simulink model "pruebaSimulink"  (Simulink 7.1)
settings: Solver=ode45  StartTime=0.0  StopTime=5  RelTol=1e-3
libraries: dsparch4 x1
settings Model: Creator=Usuario  LastModifiedBy=Usuario

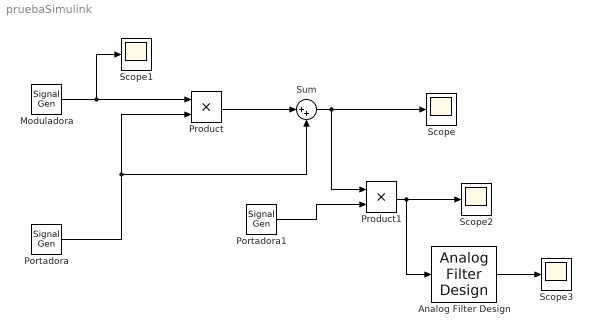
== system pruebaSimulink ==
  Analog Filter Design : dsparch4/Analog Filter Design  method=Butterworth  filttype=Lowpass  N=8  Wlo=30  Whi=80  Rp=2  Rs=40
  Moduladora : SignalGenerator
  Portadora : SignalGenerator  Frequency=10
  Portadora1 : SignalGenerator  Frequency=10
  Product : Product  OutDataType=sfix(16)  OutScaling=2^0  SampleTime=0.001  RndMeth=Zero
  Product1 : Product  OutDataType=sfix(16)  OutScaling=2^0  SampleTime=0.001  RndMeth=Zero
  Scope{,1..3} (4 alike) : Scope
      Scope2 settings: SaveName=ScopeData2
      Scope3 settings: SaveName=ScopeData3
  Sum : Sum  Inputs=|++  OutDataType=sfix(16)  OutScaling=2^0
  wires:
  Portadora/1 -> Product/2, Sum/2
  Moduladora/1 -> Product/1, Scope1/1
  Product/1 -> Sum/1
  Sum/1 -> Scope/1, Product1/1
  Product1/1 -> Scope2/1, Analog Filter Design/1
  Portadora1/1 -> Product1/2
  Analog Filter Design/1 -> Scope3/1
